simulink model "Disconnections"  (R2022a)
settings: Solver=FixedStepAuto  StartTime=0.0  StopTime=10.0  RelTol=1e-3
libraries: simulink x8
settings Model: Creator=cspt  LastModifiedBy=joser
settings SolverCC: AlgebraicLoopSolver=TrustRegion
settings DataIOCC: SaveOutput=off  ReturnWorkspaceOutputs=off
settings OptimizationCC: DefaultParameterBehavior=Inlined
settings DebuggingCC: UnconnectedInputMsg=warning  UnconnectedOutputMsg=warning  UnconnectedLineMsg=warning  SFMachineParentedDataDiag=warning  ArithmeticOperatorsInVariantConditions=warning
settings SFSimCC: SimUseLocalCustomCode=off  CustomCodeUndefinedFunction=UseInterfaceOnly
settings RTWCC: Description=INTECRIO Real-Time Target  SystemTargetFile=irt.tlc  TemplateMakefile=irt_default_tmf  RTWUseLocalCustomCode=off
settings STFCustomTargetCC: TargetLangStandard=C99 (ISO)  UtilityFuncGeneration=Shared location  MatFileLogging=on  SystemTargetFile=irt.tlc
settings GRTTargetCC: UtilityFuncGeneration=Shared location  ParMdlRefBuildCompliant=off  CompOptLevelCompliant=off  ConcurrentExecutionCompliant=off  CombineOutputUpdateFcns=off  CPPClassGenCompliant=off  GRTInterface=on  UseToolchainInfoCompliant=off  GenerateASAP2=on

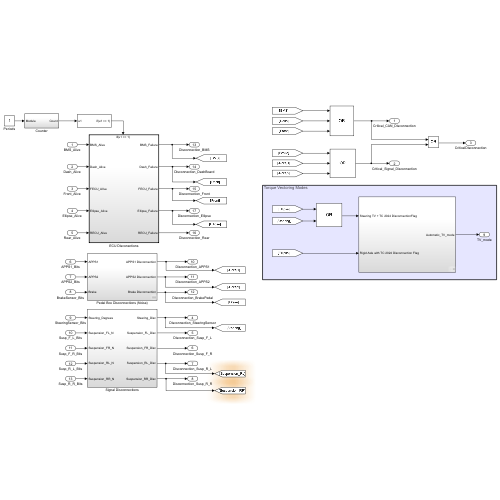
[thumbnail: Simulink's stored preview of the top-level diagram]
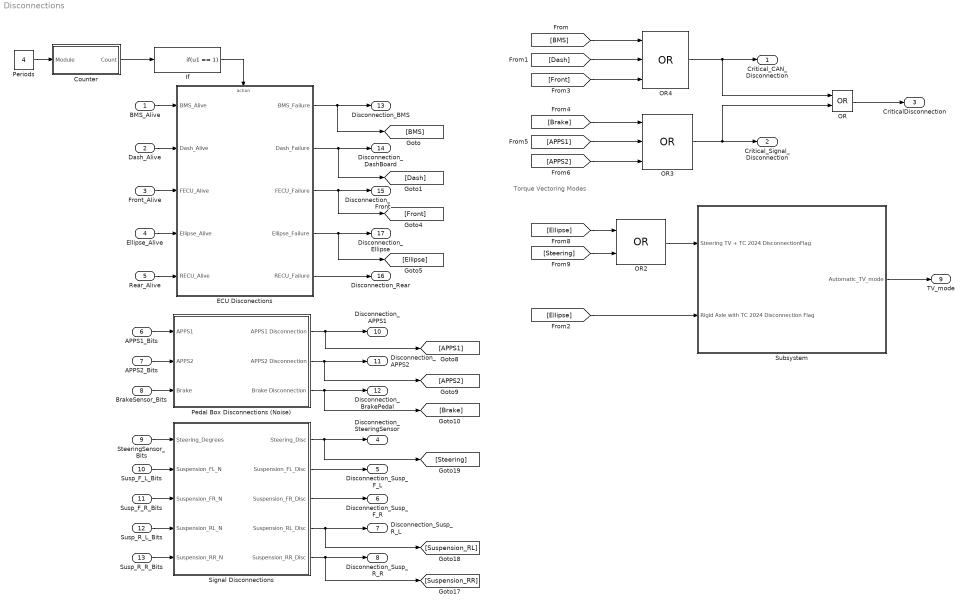
== system Disconnections ==
  note: Torque Vectoring Modes
  BMS_Alive : Inport
  Dash_Alive : Inport  Port=2
  Front_Alive : Inport  Port=3
  Ellipse_Alive : Inport  Port=4
  Rear_Alive : Inport  Port=5
  APPS1_Bits : Inport  Port=6
  APPS2_Bits : Inport  Port=7
  BrakeSensor_Bits : Inport  Port=8
  SteeringSensor_Bits : Inport  Port=9
  Susp_F_L_Bits : Inport  Port=10
  Susp_F_R_Bits : Inport  Port=11
  Susp_R_L_Bits : Inport  Port=12
  Susp_R_R_Bits : Inport  Port=13
  Counter : Subsystem
  ECU Disconections : Subsystem
  If : If  IfExpression=u1 == 1  ShowElse=off
  OR : Logic  Operator=OR  AllPortsSameDT=off  OutDataTypeStr=boolean
  OR2 : Logic  Operator=OR  AllPortsSameDT=off  OutDataTypeStr=boolean
  OR3 : Logic  Operator=OR  Inputs=3  AllPortsSameDT=off  OutDataTypeStr=boolean
  OR4 : Logic  Operator=OR  Inputs=3  AllPortsSameDT=off  OutDataTypeStr=boolean
  Pedal Box Disconnections (Noise) : Subsystem
  Periods : Constant  Value=4
  Signal Disconnections : Subsystem
  Subsystem : Subsystem
  Critical_CAN_Disconnection : Outport  VectorParamsAs1DForOutWhenUnconnected=off
  Critical_Signal_Disconnection : Outport  Port=2  VectorParamsAs1DForOutWhenUnconnected=off
  CriticalDisconnection : Outport  Port=3  VectorParamsAs1DForOutWhenUnconnected=off
  Disconnection_SteeringSensor : Outport  Port=4  VectorParamsAs1DForOutWhenUnconnected=off
  Disconnection_Susp_F_L : Outport  Port=5  VectorParamsAs1DForOutWhenUnconnected=off
  Disconnection_Susp_F_R : Outport  Port=6  VectorParamsAs1DForOutWhenUnconnected=off
  Disconnection_Susp_R_L : Outport  Port=7  VectorParamsAs1DForOutWhenUnconnected=off
  Disconnection_Susp_R_R : Outport  Port=8  VectorParamsAs1DForOutWhenUnconnected=off
  TV_mode : Outport  Port=9  VectorParamsAs1DForOutWhenUnconnected=off
  Disconnection_APPS1 : Outport  Port=10  VectorParamsAs1DForOutWhenUnconnected=off
  Disconnection_APPS2 : Outport  Port=11  VectorParamsAs1DForOutWhenUnconnected=off
  Disconnection_BrakePedal : Outport  Port=12  VectorParamsAs1DForOutWhenUnconnected=off
  Disconnection_BMS : Outport  Port=13  VectorParamsAs1DForOutWhenUnconnected=off
  Disconnection_DashBoard : Outport  Port=14  VectorParamsAs1DForOutWhenUnconnected=off
  Disconnection_Front : Outport  Port=15  VectorParamsAs1DForOutWhenUnconnected=off
  Disconnection_Rear : Outport  Port=16  VectorParamsAs1DForOutWhenUnconnected=off
  Disconnection_Ellipse : Outport  Port=17  VectorParamsAs1DForOutWhenUnconnected=off
  wires:
  [Dash] -> OR4/2
  [BMS] -> OR4/1
  [Brake] -> OR3/1
  [APPS1] -> OR3/2
  OR3/1 -> OR/2, Critical_Signal_Disconnection/1
  [APPS2] -> OR3/3
  OR/1 -> CriticalDisconnection/1
  OR4/1 -> OR/1, Critical_CAN_Disconnection/1
  Signal Disconnections/2(Suspension_FL_Disc) -> Disconnection_Susp_F_L/1
  Susp_R_L_Bits/1 -> Signal Disconnections/4(Suspension_RL_N)
  Signal Disconnections/5(Suspension_RR_Disc) -> Disconnection_Susp_R_R/1, [Suspension_RR]
  Susp_R_R_Bits/1 -> Signal Disconnections/5(Suspension_RR_N)
  Signal Disconnections/3(Suspension_FR_Disc) -> Disconnection_Susp_F_R/1
  Susp_F_R_Bits/1 -> Signal Disconnections/3(Suspension_FR_N)
  Susp_F_L_Bits/1 -> Signal Disconnections/2(Suspension_FL_N)
  SteeringSensor_Bits/1 -> Signal Disconnections/1(Steering_Degrees)
  [Steering] -> OR2/2
  OR2/1 -> Subsystem/1(Steering TV + TC 2024 DisconnectionFlag)
  Subsystem/1(Automatic_TV_mode) -> TV_mode/1
  [Ellipse] -> OR2/1
  Signal Disconnections/1(Steering_Disc) -> Disconnection_SteeringSensor/1, [Steering]
  Signal Disconnections/4(Suspension_RL_Disc) -> [Suspension_RL], Disconnection_Susp_R_L/1
  [Front] -> OR4/3
  [Ellipse] -> Subsystem/2(Rigid Axle with TC 2024 Disconnection Flag)
  Pedal Box Disconnections (Noise)/2(APPS2 Disconnection) -> Disconnection_APPS2/1, [APPS2]
  APPS2_Bits/1 -> Pedal Box Disconnections (Noise)/2(APPS2)
  APPS1_Bits/1 -> Pedal Box Disconnections (Noise)/1(APPS1)
  BrakeSensor_Bits/1 -> Pedal Box Disconnections (Noise)/3(Brake)
  Pedal Box Disconnections (Noise)/1(APPS1 Disconnection) -> [APPS1], Disconnection_APPS1/1
  Pedal Box Disconnections (Noise)/3(Brake Disconnection) -> Disconnection_BrakePedal/1, [Brake]
  Front_Alive/1 -> ECU Disconections/3(FECU_Alive)
  BMS_Alive/1 -> ECU Disconections/1(BMS_Alive)
  Dash_Alive/1 -> ECU Disconections/2(Dash_Alive)
  ECU Disconections/4(Ellipse_Failure) -> [Ellipse], Disconnection_Ellipse/1
  Ellipse_Alive/1 -> ECU Disconections/4(Ellipse_Alive)
  Rear_Alive/1 -> ECU Disconections/5(RECU_Alive)
  If/1 -> ECU Disconections/Action
  ECU Disconections/2(Dash_Failure) -> [Dash], Disconnection_DashBoard/1
  ECU Disconections/1(BMS_Failure) -> [BMS], Disconnection_BMS/1
  ECU Disconections/3(FECU_Failure) -> [Front], Disconnection_Front/1
  Counter/1(Count) -> If/1
  ECU Disconections/5(RECU_Failure) -> Disconnection_Rear/1
  Periods/1 -> Counter/1(Module)

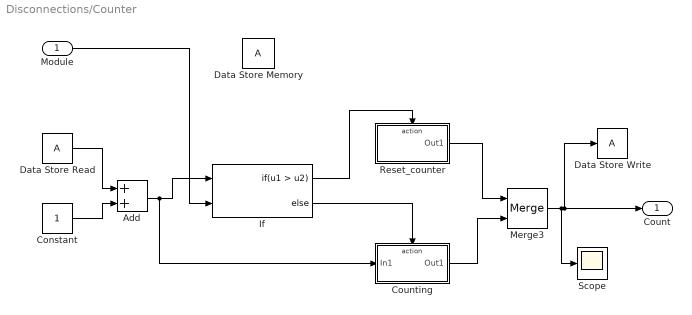
== system Disconnections/Counter ==
  Module : Inport
  Add : Sum
  Constant : Constant
  Counting : Subsystem  TreatAsAtomicUnit=on
  Data Store Memory : DataStoreMemory  ReadBeforeWriteMsg=warning  WriteAfterWriteMsg=warning  WriteAfterReadMsg=warning  ShowAdditionalParam=off
  Data Store Read : DataStoreRead  IndexOptions=Index vector (dialog)  Indices=1  OutputSizes=1
  Data Store Write : DataStoreWrite  IndexOptions=Index vector (dialog)  Indices=1  OutputSizes=1
  If : If  NumInputs=2  IfExpression=u1 > u2
  Merge3 : Merge
  Reset_counter : Subsystem  TreatAsAtomicUnit=on
  Scope : Scope
  Count : Outport  VectorParamsAs1DForOutWhenUnconnected=off
  wires:
  Data Store Read/1 -> Add/1
  Constant/1 -> Add/2
  Add/1 -> If/1, Counting/1(In1)
  If/1 -> Reset_counter/Action
  If/2 -> Counting/Action
  Reset_counter/1(Out1) -> Merge3/1
  Counting/1(Out1) -> Merge3/2
  Module/1 -> If/2
  Merge3/1 -> Scope/1, Data Store Write/1, Count/1

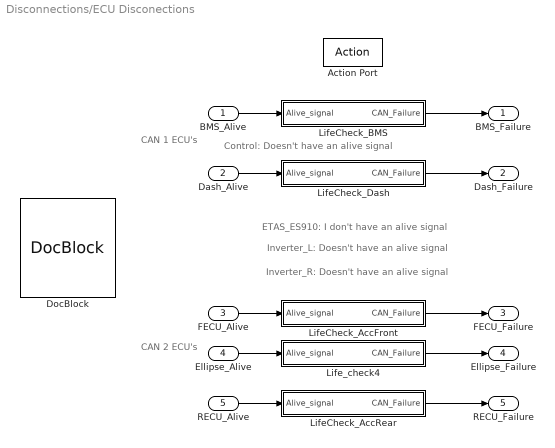
== system Disconnections/ECU Disconections ==
  note: ETAS_ES910: I don't have an alive signal
  note: Control: Doesn't have an alive signal
  note: CAN 1
      | ECU's
  note: Inverter_L: Doesn't have an alive signal
  note: Inverter_R: Doesn't have an alive signal
  note: CAN 2
      | ECU's
  BMS_Alive : Inport
  Dash_Alive : Inport  Port=2
  FECU_Alive : Inport  Port=3
  Ellipse_Alive : Inport  Port=4
  RECU_Alive : Inport  Port=5
  Action Port : ActionPort  ActionPortLabel=if(u1 == 1)
  DocBlock : simulink/Model-Wide Utilities/DocBlock  DocumentType=Text
      content=|
      | The Alive signal is sent and updated every 4 synchronisms (25ms x 4 = 100ms).
      | The Ellipse uses a counter (since the sensor is powered up, keeps going up).
      |
      | This is a Network Management Module. It takes all the alive signals of the ECU's and check if they are "alive".
      | All the ECU's for each CAN database have been extracted and listed. Some ECU's do not have an alive signal.
      |
      | Each LifeCheck generates a signal that indicate if the ECU has been disconnected.
      | OK -> 0
      | Disconnected -> 1
      |
      | The important thing about the ECU disconnection is that the ECU stopped
      | working, not the time it hasn't been working (we check a disconnection
      | every 100ms).
      |
      | There's an error -> directly ECU disconnection
  LifeCheck_AccFront : Subsystem
  LifeCheck_AccRear : Subsystem
  LifeCheck_BMS : Subsystem
  LifeCheck_Dash : Subsystem
  Life_check4 : Subsystem
  BMS_Failure : Outport  VectorParamsAs1DForOutWhenUnconnected=off
  Dash_Failure : Outport  Port=2  VectorParamsAs1DForOutWhenUnconnected=off
  FECU_Failure : Outport  Port=3  VectorParamsAs1DForOutWhenUnconnected=off
  Ellipse_Failure : Outport  Port=4  VectorParamsAs1DForOutWhenUnconnected=off
  RECU_Failure : Outport  Port=5  VectorParamsAs1DForOutWhenUnconnected=off
  wires:
  Life_check4/1(CAN_Failure) -> Ellipse_Failure/1
  Ellipse_Alive/1 -> Life_check4/1(Alive_signal)
  LifeCheck_AccFront/1(CAN_Failure) -> FECU_Failure/1
  LifeCheck_Dash/1(CAN_Failure) -> Dash_Failure/1
  Dash_Alive/1 -> LifeCheck_Dash/1(Alive_signal)
  LifeCheck_BMS/1(CAN_Failure) -> BMS_Failure/1
  FECU_Alive/1 -> LifeCheck_AccFront/1(Alive_signal)
  BMS_Alive/1 -> LifeCheck_BMS/1(Alive_signal)
  LifeCheck_AccRear/1(CAN_Failure) -> RECU_Failure/1
  RECU_Alive/1 -> LifeCheck_AccRear/1(Alive_signal)

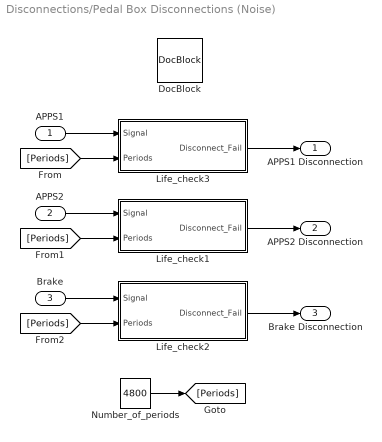
== system Disconnections/Pedal Box Disconnections (Noise) ==
  APPS1 : Inport
  APPS2 : Inport  Port=2
  Brake : Inport  Port=3
  DocBlock : simulink/Model-Wide Utilities/DocBlock  DocumentType=Text
      content=|
      | The 'Disconnections' Simulink module is computed every 25ms by the ETAS.
      |
      | A PedalBox sensor is considered disconnected if the same value is obtained
      | from it for more than X seconds:
      | 0,025sec (ETAS Sync) * 4800 periods ('Periods' constant) = X seconds
      |
      | This type of disconnection checks if there has been an error for more than
      | X seconds: STARTS counting since that first 'error' output. The important
      | thing about PedalBox disconnections is the time the signal has been
      | disconnected, that's why we do it after checking the error (not apart like
      | the ECU disconnections).
      |
      | There's a an error -> Start counting errors -> Errors persist through X
      | periods -> PedalBox disconnection
  Life_check1 : Subsystem
  Life_check2 : Subsystem
  Life_check3 : Subsystem
  Number_of_periods : Constant  Value=4800
  APPS1 Disconnection : Outport  VectorParamsAs1DForOutWhenUnconnected=off
  APPS2 Disconnection : Outport  Port=2  VectorParamsAs1DForOutWhenUnconnected=off
  Brake Disconnection : Outport  Port=3  VectorParamsAs1DForOutWhenUnconnected=off
  wires:
  Brake/1 -> Life_check2/1(Signal)
  APPS2/1 -> Life_check1/1(Signal)
  APPS1/1 -> Life_check3/1(Signal)
  Life_check3/1(Disconnect_Fail) -> APPS1 Disconnection/1
  Life_check1/1(Disconnect_Fail) -> APPS2 Disconnection/1
  Life_check2/1(Disconnect_Fail) -> Brake Disconnection/1
  Number_of_periods/1 -> [Periods]
  [Periods] -> Life_check2/2(Periods)
  [Periods] -> Life_check1/2(Periods)
  [Periods] -> Life_check3/2(Periods)

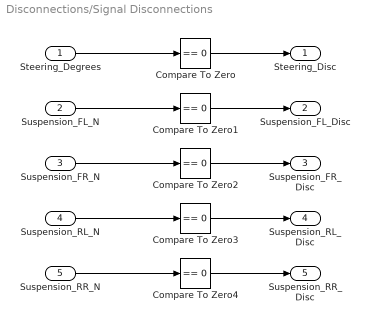
== system Disconnections/Signal Disconnections ==
  Steering_Degrees : Inport
  Suspension_FL_N : Inport  Port=2
  Suspension_FR_N : Inport  Port=3
  Suspension_RL_N : Inport  Port=4
  Suspension_RR_N : Inport  Port=5
  Compare To Zero{,1..4} (5 alike) : simulink/Logic and Bit Operations/Compare To Zero  relop===  OutDataTypeStr=uint8
  Steering_Disc : Outport  VectorParamsAs1DForOutWhenUnconnected=off
  Suspension_FL_Disc : Outport  Port=2  VectorParamsAs1DForOutWhenUnconnected=off
  Suspension_FR_Disc : Outport  Port=3  VectorParamsAs1DForOutWhenUnconnected=off
  Suspension_RL_Disc : Outport  Port=4  VectorParamsAs1DForOutWhenUnconnected=off
  Suspension_RR_Disc : Outport  Port=5  VectorParamsAs1DForOutWhenUnconnected=off
  wires:
  Compare To Zero2/1 -> Suspension_FR_Disc/1
  Suspension_FR_N/1 -> Compare To Zero2/1
  Compare To Zero3/1 -> Suspension_RL_Disc/1
  Compare To Zero1/1 -> Suspension_FL_Disc/1
  Suspension_RR_N/1 -> Compare To Zero4/1
  Suspension_FL_N/1 -> Compare To Zero1/1
  Suspension_RL_N/1 -> Compare To Zero3/1
  Compare To Zero/1 -> Steering_Disc/1
  Steering_Degrees/1 -> Compare To Zero/1
  Compare To Zero4/1 -> Suspension_RR_Disc/1

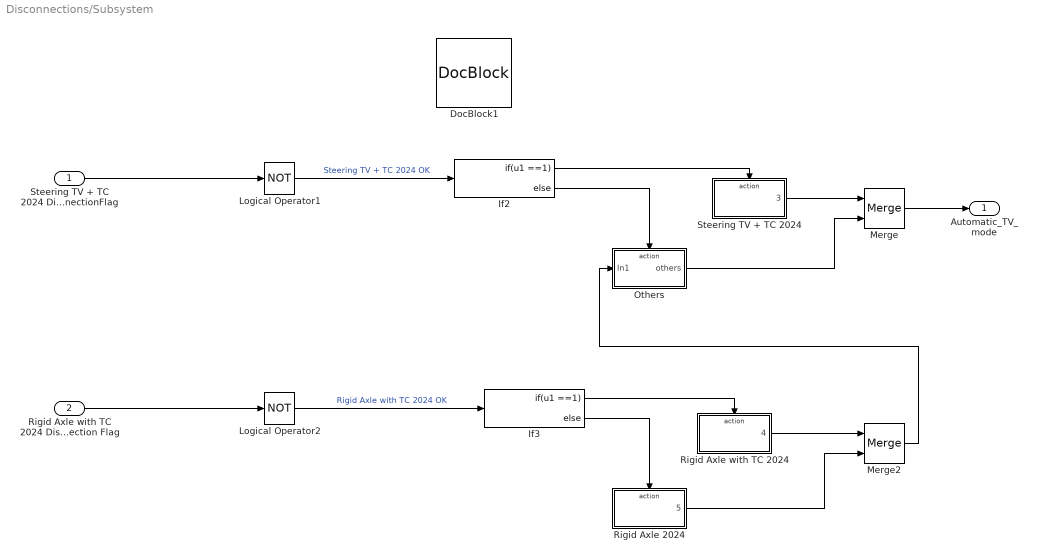
== system Disconnections/Subsystem ==
  Steering TV + TC 2024 DisconnectionFlag : Inport
  Rigid Axle with TC 2024 Disconnection Flag : Inport  Port=2
  DocBlock1 : simulink/Model-Wide Utilities/DocBlock  DocumentType=Text
      content=|
      | Checking for APPS, Brake etc... would be redundant since they are
      | critical disconnections and the car will enter to a stop state.
  If2 : If  IfExpression=u1 ==1
  If3 : If  IfExpression=u1 ==1
  Logical Operator1 : Logic  Operator=NOT  AllPortsSameDT=off  OutDataTypeStr=boolean
  Logical Operator2 : Logic  Operator=NOT  AllPortsSameDT=off  OutDataTypeStr=boolean
  Merge : Merge
  Merge2 : Merge
  "Others " : Subsystem  TreatAsAtomicUnit=on
  Rigid Axle 2024 : Subsystem  TreatAsAtomicUnit=on
  Rigid Axle with TC 2024 : Subsystem  TreatAsAtomicUnit=on
  Steering TV + TC 2024 : Subsystem  TreatAsAtomicUnit=on
  Automatic_TV_mode : Outport  VectorParamsAs1DForOutWhenUnconnected=off
  wires:
  Logical Operator2/1 -> If3/1  "Rigid Axle with TC 2024 OK"
  "Others "/1(others) -> Merge/2
  Steering TV + TC 2024/1(3) -> Merge/1
  Steering TV + TC 2024 DisconnectionFlag/1 -> Logical Operator1/1
  Logical Operator1/1 -> If2/1  "Steering TV + TC 2024 OK"
  Rigid Axle with TC 2024 Disconnection Flag/1 -> Logical Operator2/1
  If2/2 -> "Others "/Action
  If2/1 -> Steering TV + TC 2024/Action
  Rigid Axle 2024/1(5) -> Merge2/2
  Merge2/1 -> "Others "/1(In1)
  If3/2 -> Rigid Axle 2024/Action
  If3/1 -> Rigid Axle with TC 2024/Action
  Rigid Axle with TC 2024/1(4) -> Merge2/1
  Merge/1 -> Automatic_TV_mode/1

== system Disconnections/Counter/Counting ==
  In1 : Inport
  Action Port : ActionPort
  Out1 : Outport  VectorParamsAs1DForOutWhenUnconnected=off
  wires:
  In1/1 -> Out1/1

== system Disconnections/Counter/Reset_counter ==
  Action Port : ActionPort
  Constant : Constant
  Out1 : Outport  VectorParamsAs1DForOutWhenUnconnected=off
  wires:
  Constant/1 -> Out1/1

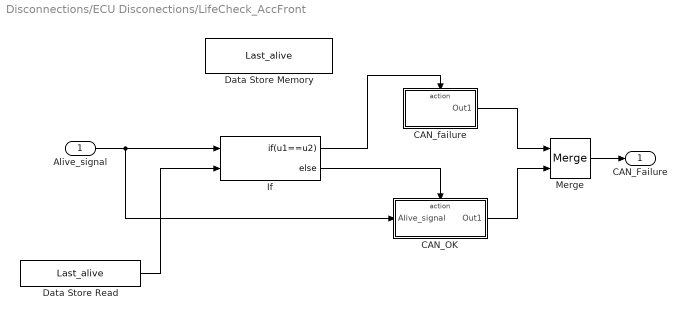
== system Disconnections/ECU Disconections/LifeCheck_AccFront ==
  Alive_signal : Inport
  CAN_OK : Subsystem  TreatAsAtomicUnit=on
  CAN_failure : Subsystem  TreatAsAtomicUnit=on
  Data Store Memory : DataStoreMemory  DataStoreName=Last_alive  ReadBeforeWriteMsg=warning  WriteAfterWriteMsg=warning  WriteAfterReadMsg=warning  ShowAdditionalParam=off
  Data Store Read : DataStoreRead  DataStoreName=Last_alive  IndexOptions=Index vector (dialog)  Indices=1  OutputSizes=1
  If : If  NumInputs=2  IfExpression=u1==u2
  Merge : Merge
  CAN_Failure : Outport  VectorParamsAs1DForOutWhenUnconnected=off
  wires:
  Data Store Read/1 -> If/2
  If/1 -> CAN_failure/Action
  If/2 -> CAN_OK/Action
  CAN_failure/1(Out1) -> Merge/1
  CAN_OK/1(Out1) -> Merge/2
  Merge/1 -> CAN_Failure/1
  Alive_signal/1 -> CAN_OK/1(Alive_signal), If/1

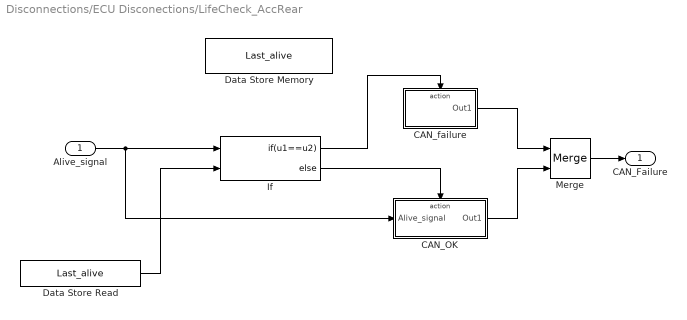
== system Disconnections/ECU Disconections/LifeCheck_AccRear ==
  Alive_signal : Inport
  CAN_OK : Subsystem  TreatAsAtomicUnit=on
  CAN_failure : Subsystem  TreatAsAtomicUnit=on
  Data Store Memory : DataStoreMemory  DataStoreName=Last_alive  ReadBeforeWriteMsg=warning  WriteAfterWriteMsg=warning  WriteAfterReadMsg=warning  ShowAdditionalParam=off
  Data Store Read : DataStoreRead  DataStoreName=Last_alive  IndexOptions=Index vector (dialog)  Indices=1  OutputSizes=1
  If : If  NumInputs=2  IfExpression=u1==u2
  Merge : Merge
  CAN_Failure : Outport  VectorParamsAs1DForOutWhenUnconnected=off
  wires:
  Data Store Read/1 -> If/2
  If/1 -> CAN_failure/Action
  If/2 -> CAN_OK/Action
  CAN_failure/1(Out1) -> Merge/1
  CAN_OK/1(Out1) -> Merge/2
  Merge/1 -> CAN_Failure/1
  Alive_signal/1 -> CAN_OK/1(Alive_signal), If/1

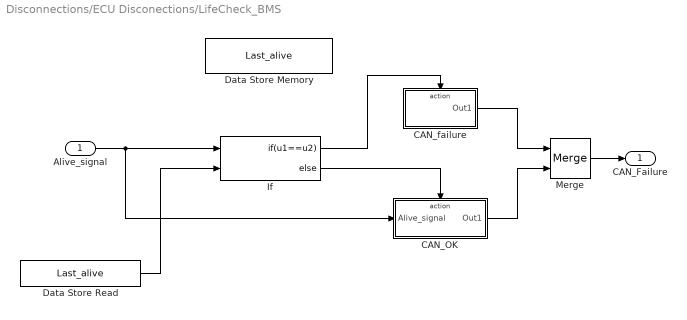
== system Disconnections/ECU Disconections/LifeCheck_BMS ==
  Alive_signal : Inport
  CAN_OK : Subsystem  TreatAsAtomicUnit=on
  CAN_failure : Subsystem  TreatAsAtomicUnit=on
  Data Store Memory : DataStoreMemory  DataStoreName=Last_alive  ReadBeforeWriteMsg=warning  WriteAfterWriteMsg=warning  WriteAfterReadMsg=warning  ShowAdditionalParam=off
  Data Store Read : DataStoreRead  DataStoreName=Last_alive  IndexOptions=Index vector (dialog)  Indices=1  OutputSizes=1
  If : If  NumInputs=2  IfExpression=u1==u2
  Merge : Merge
  CAN_Failure : Outport  VectorParamsAs1DForOutWhenUnconnected=off
  wires:
  Data Store Read/1 -> If/2
  If/1 -> CAN_failure/Action
  If/2 -> CAN_OK/Action
  CAN_failure/1(Out1) -> Merge/1
  CAN_OK/1(Out1) -> Merge/2
  Merge/1 -> CAN_Failure/1
  Alive_signal/1 -> CAN_OK/1(Alive_signal), If/1

== system Disconnections/ECU Disconections/LifeCheck_Dash ==
  Alive_signal : Inport
  CAN_OK : Subsystem  TreatAsAtomicUnit=on
  CAN_failure : Subsystem  TreatAsAtomicUnit=on
  Data Store Memory : DataStoreMemory  DataStoreName=Last_alive  ReadBeforeWriteMsg=warning  WriteAfterWriteMsg=warning  WriteAfterReadMsg=warning  ShowAdditionalParam=off
  Data Store Read : DataStoreRead  DataStoreName=Last_alive  IndexOptions=Index vector (dialog)  Indices=1  OutputSizes=1
  If : If  NumInputs=2  IfExpression=u1==u2
  Merge : Merge
  CAN_Failure : Outport  VectorParamsAs1DForOutWhenUnconnected=off
  wires:
  Data Store Read/1 -> If/2
  If/1 -> CAN_failure/Action
  If/2 -> CAN_OK/Action
  CAN_failure/1(Out1) -> Merge/1
  CAN_OK/1(Out1) -> Merge/2
  Merge/1 -> CAN_Failure/1
  Alive_signal/1 -> CAN_OK/1(Alive_signal), If/1

== system Disconnections/ECU Disconections/Life_check4 ==
  Alive_signal : Inport
  CAN_OK : Subsystem  TreatAsAtomicUnit=on
  CAN_failure : Subsystem  TreatAsAtomicUnit=on
  Data Store Memory : DataStoreMemory  DataStoreName=Last_alive  ReadBeforeWriteMsg=warning  WriteAfterWriteMsg=warning  WriteAfterReadMsg=warning  ShowAdditionalParam=off
  Data Store Read : DataStoreRead  DataStoreName=Last_alive  IndexOptions=Index vector (dialog)  Indices=1  OutputSizes=1
  If : If  NumInputs=2  IfExpression=u1==u2
  Merge : Merge
  CAN_Failure : Outport  VectorParamsAs1DForOutWhenUnconnected=off
  wires:
  Data Store Read/1 -> If/2
  If/1 -> CAN_failure/Action
  If/2 -> CAN_OK/Action
  CAN_failure/1(Out1) -> Merge/1
  CAN_OK/1(Out1) -> Merge/2
  Merge/1 -> CAN_Failure/1
  Alive_signal/1 -> CAN_OK/1(Alive_signal), If/1

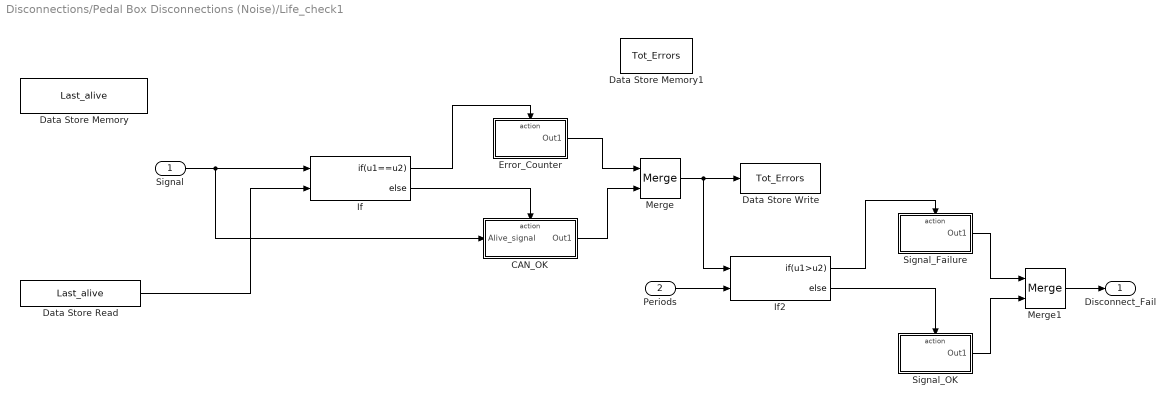
== system Disconnections/Pedal Box Disconnections (Noise)/Life_check1 ==
  Signal : Inport
  Periods : Inport  Port=2
  CAN_OK : Subsystem  TreatAsAtomicUnit=on
  Data Store Memory : DataStoreMemory  DataStoreName=Last_alive  ReadBeforeWriteMsg=warning  WriteAfterWriteMsg=warning  WriteAfterReadMsg=warning  ShowAdditionalParam=off
  Data Store Memory1 : DataStoreMemory  DataStoreName=Tot_Errors  ReadBeforeWriteMsg=warning  WriteAfterWriteMsg=warning  WriteAfterReadMsg=warning  ShowAdditionalParam=off
  Data Store Read : DataStoreRead  DataStoreName=Last_alive  IndexOptions=Index vector (dialog)  Indices=1  OutputSizes=1
  Data Store Write : DataStoreWrite  DataStoreName=Tot_Errors  IndexOptions=Index vector (dialog)  Indices=1  OutputSizes=1
  Error_Counter : Subsystem  TreatAsAtomicUnit=on
  If : If  NumInputs=2  IfExpression=u1==u2
  If2 : If  NumInputs=2  IfExpression=u1>u2
  Merge : Merge
  Merge1 : Merge
  Signal_Failure : Subsystem  TreatAsAtomicUnit=on
  Signal_OK : Subsystem  TreatAsAtomicUnit=on
  Disconnect_Fail : Outport  VectorParamsAs1DForOutWhenUnconnected=off
  wires:
  Data Store Read/1 -> If/2
  If/2 -> CAN_OK/Action
  CAN_OK/1(Out1) -> Merge/2
  Signal/1 -> CAN_OK/1(Alive_signal), If/1
  If/1 -> Error_Counter/Action
  Error_Counter/1(Out1) -> Merge/1
  Signal_Failure/1(Out1) -> Merge1/1
  Signal_OK/1(Out1) -> Merge1/2
  Merge1/1 -> Disconnect_Fail/1
  If2/2 -> Signal_OK/Action
  Periods/1 -> If2/2
  If2/1 -> Signal_Failure/Action
  Merge/1 -> If2/1, Data Store Write/1

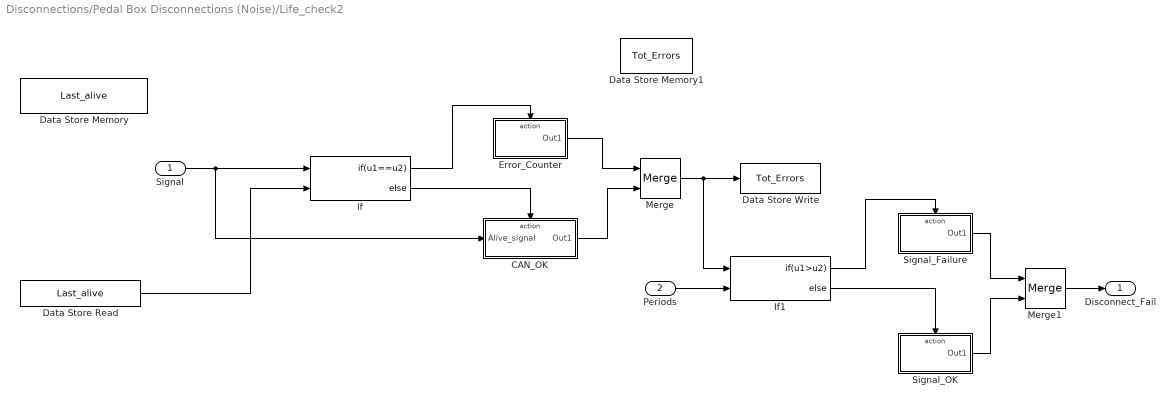
== system Disconnections/Pedal Box Disconnections (Noise)/Life_check2 ==
  Signal : Inport
  Periods : Inport  Port=2
  CAN_OK : Subsystem  TreatAsAtomicUnit=on
  Data Store Memory : DataStoreMemory  DataStoreName=Last_alive  ReadBeforeWriteMsg=warning  WriteAfterWriteMsg=warning  WriteAfterReadMsg=warning  ShowAdditionalParam=off
  Data Store Memory1 : DataStoreMemory  DataStoreName=Tot_Errors  ReadBeforeWriteMsg=warning  WriteAfterWriteMsg=warning  WriteAfterReadMsg=warning  ShowAdditionalParam=off
  Data Store Read : DataStoreRead  DataStoreName=Last_alive  IndexOptions=Index vector (dialog)  Indices=1  OutputSizes=1
  Data Store Write : DataStoreWrite  DataStoreName=Tot_Errors  IndexOptions=Index vector (dialog)  Indices=1  OutputSizes=1
  Error_Counter : Subsystem  TreatAsAtomicUnit=on
  If : If  NumInputs=2  IfExpression=u1==u2
  If1 : If  NumInputs=2  IfExpression=u1>u2
  Merge : Merge
  Merge1 : Merge
  Signal_Failure : Subsystem  TreatAsAtomicUnit=on
  Signal_OK : Subsystem  TreatAsAtomicUnit=on
  Disconnect_Fail : Outport  VectorParamsAs1DForOutWhenUnconnected=off
  wires:
  Data Store Read/1 -> If/2
  If/2 -> CAN_OK/Action
  CAN_OK/1(Out1) -> Merge/2
  Signal/1 -> CAN_OK/1(Alive_signal), If/1
  If/1 -> Error_Counter/Action
  Error_Counter/1(Out1) -> Merge/1
  Signal_Failure/1(Out1) -> Merge1/1
  Signal_OK/1(Out1) -> Merge1/2
  Merge1/1 -> Disconnect_Fail/1
  If1/2 -> Signal_OK/Action
  Periods/1 -> If1/2
  If1/1 -> Signal_Failure/Action
  Merge/1 -> If1/1, Data Store Write/1

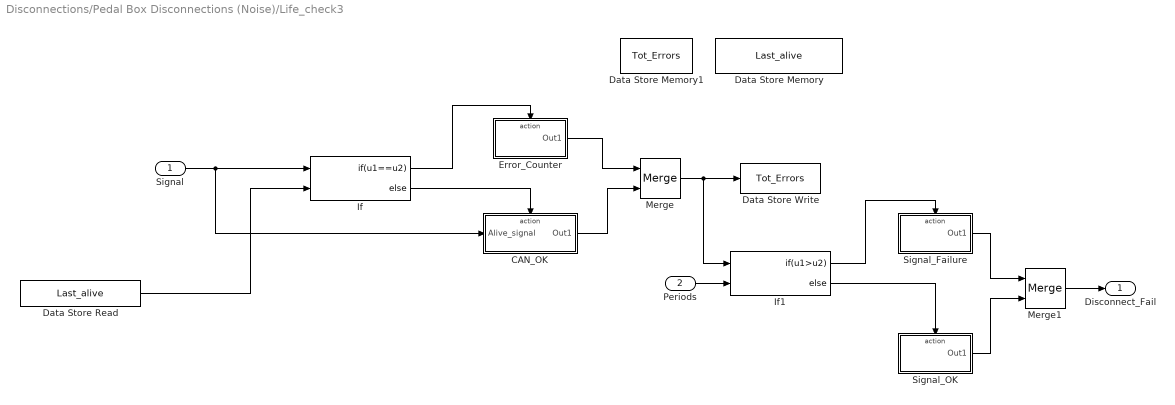
== system Disconnections/Pedal Box Disconnections (Noise)/Life_check3 ==
  Signal : Inport
  Periods : Inport  Port=2
  CAN_OK : Subsystem  TreatAsAtomicUnit=on
  Data Store Memory : DataStoreMemory  DataStoreName=Last_alive  ReadBeforeWriteMsg=warning  WriteAfterWriteMsg=warning  WriteAfterReadMsg=warning  ShowAdditionalParam=off
  Data Store Memory1 : DataStoreMemory  DataStoreName=Tot_Errors  ReadBeforeWriteMsg=warning  WriteAfterWriteMsg=warning  WriteAfterReadMsg=warning  ShowAdditionalParam=off
  Data Store Read : DataStoreRead  DataStoreName=Last_alive  IndexOptions=Index vector (dialog)  Indices=1  OutputSizes=1
  Data Store Write : DataStoreWrite  DataStoreName=Tot_Errors  IndexOptions=Index vector (dialog)  Indices=1  OutputSizes=1
  Error_Counter : Subsystem  TreatAsAtomicUnit=on
  If : If  NumInputs=2  IfExpression=u1==u2
  If1 : If  NumInputs=2  IfExpression=u1>u2
  Merge : Merge
  Merge1 : Merge
  Signal_Failure : Subsystem  TreatAsAtomicUnit=on
  Signal_OK : Subsystem  TreatAsAtomicUnit=on
  Disconnect_Fail : Outport  VectorParamsAs1DForOutWhenUnconnected=off
  wires:
  Data Store Read/1 -> If/2
  If/2 -> CAN_OK/Action
  CAN_OK/1(Out1) -> Merge/2
  Merge/1 -> If1/1, Data Store Write/1
  Signal/1 -> CAN_OK/1(Alive_signal), If/1
  If/1 -> Error_Counter/Action
  Error_Counter/1(Out1) -> Merge/1
  If1/1 -> Signal_Failure/Action
  If1/2 -> Signal_OK/Action
  Signal_Failure/1(Out1) -> Merge1/1
  Signal_OK/1(Out1) -> Merge1/2
  Merge1/1 -> Disconnect_Fail/1
  Periods/1 -> If1/2

== system Disconnections/Subsystem/Others  ==
  In1 : Inport
  Action Port : ActionPort  ActionPortLabel=else
  others : Outport  VectorParamsAs1DForOutWhenUnconnected=off
  wires:
  In1/1 -> others/1

== system Disconnections/Subsystem/Rigid Axle 2024 ==
  Action Port : ActionPort  ActionPortLabel=else
  Constant : Constant  Value=5
  5 : Outport  VectorParamsAs1DForOutWhenUnconnected=off
  wires:
  Constant/1 -> 5/1

== system Disconnections/Subsystem/Rigid Axle with TC 2024 ==
  Action Port : ActionPort  ActionPortLabel=if(u1 ==1)
  Constant : Constant  Value=4
  4 : Outport  VectorParamsAs1DForOutWhenUnconnected=off
  wires:
  Constant/1 -> 4/1

== system Disconnections/Subsystem/Steering TV + TC 2024 ==
  Action Port : ActionPort  ActionPortLabel=if(u1 ==1)
  Constant : Constant  Value=3
  3 : Outport  VectorParamsAs1DForOutWhenUnconnected=off
  wires:
  Constant/1 -> 3/1

== system Disconnections/ECU Disconections/LifeCheck_AccFront/CAN_OK ==
  Alive_signal : Inport
  Action Port : ActionPort
  Constant : Constant  Value=0
  Data Store Write : DataStoreWrite  DataStoreName=Last_alive  IndexOptions=Index vector (dialog)  Indices=1  OutputSizes=1
  Out1 : Outport  VectorParamsAs1DForOutWhenUnconnected=off
  wires:
  Constant/1 -> Out1/1
  Alive_signal/1 -> Data Store Write/1

== system Disconnections/ECU Disconections/LifeCheck_AccFront/CAN_failure ==
  Action Port : ActionPort
  Constant : Constant
  Out1 : Outport  VectorParamsAs1DForOutWhenUnconnected=off
  wires:
  Constant/1 -> Out1/1

== system Disconnections/ECU Disconections/LifeCheck_AccRear/CAN_OK ==
  Alive_signal : Inport
  Action Port : ActionPort
  Constant : Constant  Value=0
  Data Store Write : DataStoreWrite  DataStoreName=Last_alive  IndexOptions=Index vector (dialog)  Indices=1  OutputSizes=1
  Out1 : Outport  VectorParamsAs1DForOutWhenUnconnected=off
  wires:
  Constant/1 -> Out1/1
  Alive_signal/1 -> Data Store Write/1

== system Disconnections/ECU Disconections/LifeCheck_AccRear/CAN_failure ==
  Action Port : ActionPort
  Constant : Constant
  Out1 : Outport  VectorParamsAs1DForOutWhenUnconnected=off
  wires:
  Constant/1 -> Out1/1

== system Disconnections/ECU Disconections/LifeCheck_BMS/CAN_OK ==
  Alive_signal : Inport
  Action Port : ActionPort
  Constant : Constant  Value=0
  Data Store Write : DataStoreWrite  DataStoreName=Last_alive  IndexOptions=Index vector (dialog)  Indices=1  OutputSizes=1
  Out1 : Outport  VectorParamsAs1DForOutWhenUnconnected=off
  wires:
  Constant/1 -> Out1/1
  Alive_signal/1 -> Data Store Write/1

== system Disconnections/ECU Disconections/LifeCheck_BMS/CAN_failure ==
  Action Port : ActionPort
  Constant : Constant
  Out1 : Outport  VectorParamsAs1DForOutWhenUnconnected=off
  wires:
  Constant/1 -> Out1/1

== system Disconnections/ECU Disconections/LifeCheck_Dash/CAN_OK ==
  Alive_signal : Inport
  Action Port : ActionPort
  Constant : Constant  Value=0
  Data Store Write : DataStoreWrite  DataStoreName=Last_alive  IndexOptions=Index vector (dialog)  Indices=1  OutputSizes=1
  Out1 : Outport  VectorParamsAs1DForOutWhenUnconnected=off
  wires:
  Constant/1 -> Out1/1
  Alive_signal/1 -> Data Store Write/1

== system Disconnections/ECU Disconections/LifeCheck_Dash/CAN_failure ==
  Action Port : ActionPort
  Constant : Constant
  Out1 : Outport  VectorParamsAs1DForOutWhenUnconnected=off
  wires:
  Constant/1 -> Out1/1

== system Disconnections/ECU Disconections/Life_check4/CAN_OK ==
  Alive_signal : Inport
  Action Port : ActionPort
  Constant : Constant  Value=0
  Data Store Write : DataStoreWrite  DataStoreName=Last_alive  IndexOptions=Index vector (dialog)  Indices=1  OutputSizes=1
  Out1 : Outport  VectorParamsAs1DForOutWhenUnconnected=off
  wires:
  Constant/1 -> Out1/1
  Alive_signal/1 -> Data Store Write/1

== system Disconnections/ECU Disconections/Life_check4/CAN_failure ==
  Action Port : ActionPort
  Constant : Constant
  Out1 : Outport  VectorParamsAs1DForOutWhenUnconnected=off
  wires:
  Constant/1 -> Out1/1

== system Disconnections/Pedal Box Disconnections (Noise)/Life_check1/CAN_OK ==
  Alive_signal : Inport
  Action Port : ActionPort
  Constant : Constant  Value=0
  Data Store Write : DataStoreWrite  DataStoreName=Last_alive  IndexOptions=Index vector (dialog)  Indices=1  OutputSizes=1
  Out1 : Outport  VectorParamsAs1DForOutWhenUnconnected=off
  wires:
  Constant/1 -> Out1/1
  Alive_signal/1 -> Data Store Write/1

== system Disconnections/Pedal Box Disconnections (Noise)/Life_check1/Error_Counter ==
  Action Port : ActionPort
  Add : Sum
  Constant : Constant
  Data Store Read1 : DataStoreRead  DataStoreName=Tot_Errors  IndexOptions=Index vector (dialog)  Indices=1  OutputSizes=1
  Out1 : Outport  VectorParamsAs1DForOutWhenUnconnected=off
  wires:
  Constant/1 -> Add/2
  Data Store Read1/1 -> Add/1
  Add/1 -> Out1/1

== system Disconnections/Pedal Box Disconnections (Noise)/Life_check1/Signal_Failure ==
  Action Port : ActionPort
  Constant : Constant
  Out1 : Outport  VectorParamsAs1DForOutWhenUnconnected=off
  wires:
  Constant/1 -> Out1/1

== system Disconnections/Pedal Box Disconnections (Noise)/Life_check1/Signal_OK ==
  Action Port : ActionPort
  Constant : Constant  Value=0
  Out1 : Outport  VectorParamsAs1DForOutWhenUnconnected=off
  wires:
  Constant/1 -> Out1/1

== system Disconnections/Pedal Box Disconnections (Noise)/Life_check2/CAN_OK ==
  Alive_signal : Inport
  Action Port : ActionPort
  Constant : Constant  Value=0
  Data Store Write : DataStoreWrite  DataStoreName=Last_alive  IndexOptions=Index vector (dialog)  Indices=1  OutputSizes=1
  Out1 : Outport  VectorParamsAs1DForOutWhenUnconnected=off
  wires:
  Constant/1 -> Out1/1
  Alive_signal/1 -> Data Store Write/1

== system Disconnections/Pedal Box Disconnections (Noise)/Life_check2/Error_Counter ==
  Action Port : ActionPort
  Add : Sum
  Constant : Constant
  Data Store Read1 : DataStoreRead  DataStoreName=Tot_Errors  IndexOptions=Index vector (dialog)  Indices=1  OutputSizes=1
  Out1 : Outport  VectorParamsAs1DForOutWhenUnconnected=off
  wires:
  Constant/1 -> Add/2
  Data Store Read1/1 -> Add/1
  Add/1 -> Out1/1

== system Disconnections/Pedal Box Disconnections (Noise)/Life_check2/Signal_Failure ==
  Action Port : ActionPort
  Constant : Constant
  Out1 : Outport  VectorParamsAs1DForOutWhenUnconnected=off
  wires:
  Constant/1 -> Out1/1

== system Disconnections/Pedal Box Disconnections (Noise)/Life_check2/Signal_OK ==
  Action Port : ActionPort
  Constant : Constant  Value=0
  Out1 : Outport  VectorParamsAs1DForOutWhenUnconnected=off
  wires:
  Constant/1 -> Out1/1

== system Disconnections/Pedal Box Disconnections (Noise)/Life_check3/CAN_OK ==
  Alive_signal : Inport
  Action Port : ActionPort
  Constant : Constant  Value=0
  Data Store Write : DataStoreWrite  DataStoreName=Last_alive  IndexOptions=Index vector (dialog)  Indices=1  OutputSizes=1
  Out1 : Outport  VectorParamsAs1DForOutWhenUnconnected=off
  wires:
  Constant/1 -> Out1/1
  Alive_signal/1 -> Data Store Write/1

== system Disconnections/Pedal Box Disconnections (Noise)/Life_check3/Error_Counter ==
  Action Port : ActionPort
  Add : Sum
  Constant : Constant
  Data Store Read1 : DataStoreRead  DataStoreName=Tot_Errors  IndexOptions=Index vector (dialog)  Indices=1  OutputSizes=1
  Out1 : Outport  VectorParamsAs1DForOutWhenUnconnected=off
  wires:
  Constant/1 -> Add/2
  Data Store Read1/1 -> Add/1
  Add/1 -> Out1/1

== system Disconnections/Pedal Box Disconnections (Noise)/Life_check3/Signal_Failure ==
  Action Port : ActionPort
  Constant : Constant
  Out1 : Outport  VectorParamsAs1DForOutWhenUnconnected=off
  wires:
  Constant/1 -> Out1/1

== system Disconnections/Pedal Box Disconnections (Noise)/Life_check3/Signal_OK ==
  Action Port : ActionPort
  Constant : Constant  Value=0
  Out1 : Outport  VectorParamsAs1DForOutWhenUnconnected=off
  wires:
  Constant/1 -> Out1/1
